simulink model "Model1_Scenario2_Faulty_2020a_35"  (R2024a)
settings: Solver=FixedStepAuto  StartTime=0.0  StopTime=300  FixedStep=1e-2  RelTol=1e-3  EnableMultiTasking=on
undefined symbols (not defined in the file): sigbuilder_block
settings Model: PacingRate=0.250000  ExtModeTrigDuration=5  Creator=Arun Mistry  LastModifiedBy=airshad
settings SolverCC: AlgebraicLoopSolver=TrustRegion
settings DataIOCC: SaveFormat=Array  SaveOutput=off  SignalLogging=off  DSMLogging=off  SaveTime=off  ReturnWorkspaceOutputs=off
settings OptimizationCC: DefaultParameterBehavior=Inlined  DefaultUnderspecifiedDataType=single  EnhancedBackFolding=on  PassReuseOutputArgsAs=Individual arguments  ZeroExternalMemoryAtStartup=off  ZeroInternalMemoryAtStartup=off  MaxStackSize=64  OptimizeBlockOrder=speed  DifferentSizesBufferReuse=on  OptimizationCustomize=off  EfficientTunableParamExpr=on
settings DebuggingCC: ParameterTunabilityLossMsg=error  UnconnectedInputMsg=warning  UnconnectedOutputMsg=warning  UnconnectedLineMsg=warning
settings HardwareCC: ProdBitPerPointer=32  ProdBitPerSizeT=32  ProdBitPerPtrDiffT=32  ProdLargestAtomicInteger=Long  ProdLargestAtomicFloat=Double  ProdWordSize=32  ProdHWDeviceType=ARM Compatible->ARM Cortex
settings ModelReferenceCC: EnableRefExpFcnMdlSchedulingChecks=on
settings SFSimCC: SimParseCustomCode=off  MATLABDynamicMemAlloc=off
settings RTWCC: Description=Embedded Coder  SystemTargetFile=ert.tlc  TemplateMakefile=ert_default_tmf  Toolchain=GNU Tools for ARM Embedded Processors  GPUComputeCapability=3.5  DLArmComputeVersion=19.05
settings CodeAppCC: ForceParamTrailComments=on  IgnoreCustomStorageClasses=off  OperatorAnnotations=on  SimulinkDataObjDesc=on  SFDataObjDesc=on  InsertBlockDesc=on
settings ERTTargetCC: ERTCustomFileTemplate=example_file_process.tlc

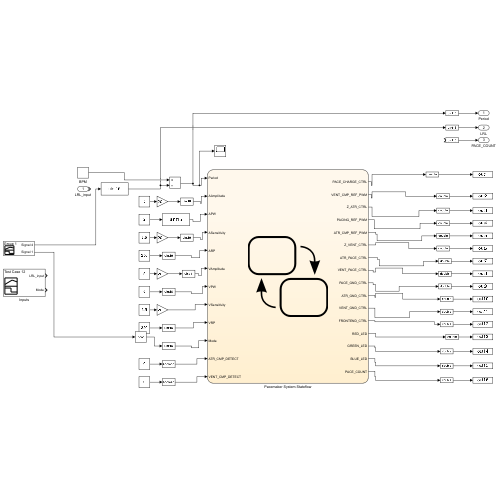
[thumbnail: Simulink's stored preview of the top-level diagram]
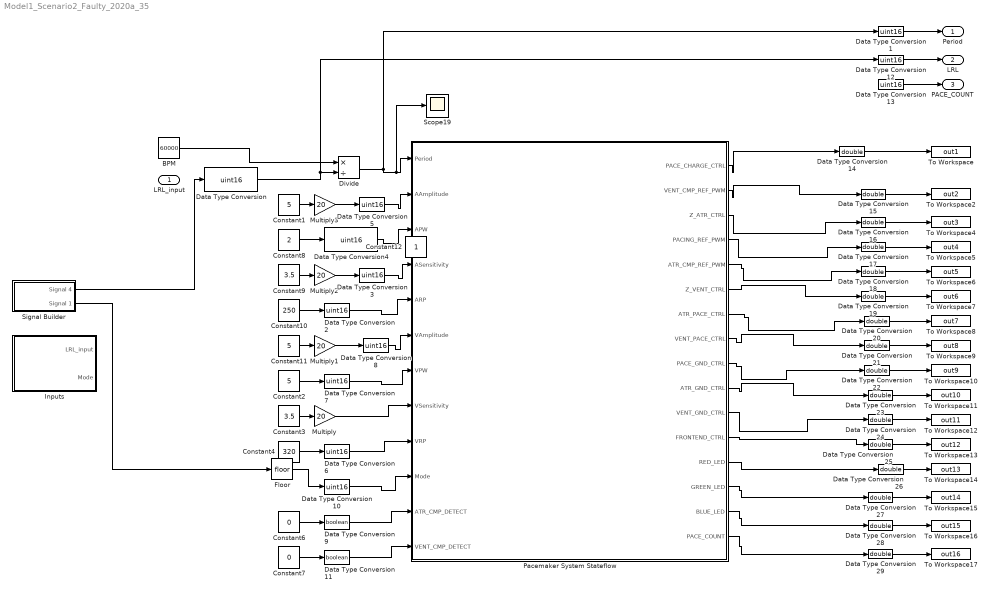
== system Model1_Scenario2_Faulty_2020a_35 ==
  LRL_input : Inport  OutDataTypeStr=double
  BPM : Constant  Value=60000
  Constant1 : Constant  Value=5
  Constant10 : Constant  Value=250
  Constant11 : Constant  Value=5
  Constant2 : Constant  Value=5
  Constant3 : Constant  Value=3.5
  Constant4 : Constant  Value=320
  Constant6 : Constant  Value=0
  Constant7 : Constant  Value=0
  Constant8 : Constant  Value=2
  Constant9 : Constant  Value=3.5
  Data Type Conversion{,1..8,10,12..13} (12 alike) : DataTypeConversion  OutDataTypeStr=uint16  SaturateOnIntegerOverflow=off  RndMeth=Floor
  Data Type Conversion11 : DataTypeConversion  OutDataTypeStr=boolean  SaturateOnIntegerOverflow=off  RndMeth=Floor
  Data Type Conversion{14..29} (16 alike) : DataTypeConversion  OutDataTypeStr=double  SaturateOnIntegerOverflow=off  RndMeth=Floor
  Data Type Conversion9 : DataTypeConversion  OutDataTypeStr=boolean  SaturateOnIntegerOverflow=off  RndMeth=Floor
  Divide : Product  Inputs=*/
  Floor : Rounding
  Inputs : Subsystem  Tag=STV Subsys  LoadFcn=sigbuilder_block('load');  StartFcn=sigbuilder_block('start');  StopFcn=sigbuilder_block('stop');  ClipboardFcn=sigbuilder_block('clipboard');  mask(Sigbuilder block){tuvar=[0:10]}
      mask init:
      | if ~strcmp(get_param(bdroot(gcb),'SimulationStatus'),'stopped'),tuvar = sigbuilder_block('maskInit'); end
      settings: CopyFcn=sigbuilder_block('copy');  DeleteFcn=sigbuilder_block('delete');  ModelCloseFcn=sigbuilder_block('modelClose');  PreSaveFcn=sigbuilder_block('preSave');  PauseFcn=sigbuilder_block('pause');  ContinueFcn=sigbuilder_block('continue');  NameChangeFcn=sigbuilder_block('namechange');  OpenFcn=sigbuilder_block('open',[50 50 520 400 ]);  CloseFcn=sigbuilder_block('close');
      mask Display: plot(0, 0, 100, 100,[2, 2, 32, 32, 2], [68, 8, 8, 68, 68],[32, 2], [38, 38], [32, 19, 2],[53, 60, 44], [32, 17, 17, 2],[16, 16, 31, 31]);txt = getActiveGroup(gcbh);text(2, 100, txt,'verticalAlignment', 'top');
  Multiply{,1..3} (4 alike) : Gain  Gain=20
  Pacemaker System Stateflow : Stateflow chart  TreatAsAtomicUnit=on
  Scope19 : Scope
  Signal Builder : Subsystem  Tag=STV Subsys  LoadFcn=sigbuilder_block('load');  StartFcn=sigbuilder_block('start');  StopFcn=sigbuilder_block('stop');  ClipboardFcn=sigbuilder_block('clipboard');  mask(Sigbuilder block){tuvar=[0:10]}
      mask help: Simulink:masks:SigbuilderBlock_MD
      mask init:
      | if ~strcmp(get_param(bdroot(gcbh),'SimulationStatus'),'stopped') tuvar = sigbuilder_block('maskInit'); end
      settings: CopyFcn=sigbuilder_block('copy');  DeleteFcn=sigbuilder_block('delete');  ModelCloseFcn=sigbuilder_block('modelClose');  PreSaveFcn=sigbuilder_block('preSave');  PauseFcn=sigbuilder_block('pause');  ContinueFcn=sigbuilder_block('continue');  NameChangeFcn=sigbuilder_block('namechange');  OpenFcn=sigbuilder_block('open',[6 26.4 948 559.8 ]);  CloseFcn=sigbuilder_block('close');
      mask Display: plot(0, 0, 100, 100,[2, 2, 32, 32, 2], [68, 8, 8, 68, 68],[32, 2], [38, 38], [32, 19, 2],[53, 60, 44], [32, 17, 17, 2],[16, 16, 31, 31]);txt = getActiveGroup(gcbh);text(2, 100, txt,'verticalAlignment', 'top');
  To Workspace : ToWorkspace  VariableName=out1  SaveFormat=Timeseries  SampleTime=-1
  To Workspace10 : ToWorkspace  VariableName=out9  SaveFormat=Timeseries  SampleTime=-1
  To Workspace11 : ToWorkspace  VariableName=out10  SaveFormat=Timeseries  SampleTime=-1
  To Workspace12 : ToWorkspace  VariableName=out11  SaveFormat=Timeseries  SampleTime=-1
  To Workspace13 : ToWorkspace  VariableName=out12  SaveFormat=Timeseries  SampleTime=-1
  To Workspace14 : ToWorkspace  VariableName=out13  SaveFormat=Timeseries  SampleTime=-1
  To Workspace15 : ToWorkspace  VariableName=out14  SaveFormat=Timeseries  SampleTime=-1
  To Workspace16 : ToWorkspace  VariableName=out15  SaveFormat=Timeseries  SampleTime=-1
  To Workspace17 : ToWorkspace  VariableName=out16  SaveFormat=Timeseries  SampleTime=-1
  To Workspace2 : ToWorkspace  VariableName=out2  SaveFormat=Timeseries  SampleTime=-1
  To Workspace4 : ToWorkspace  VariableName=out3  SaveFormat=Timeseries  SampleTime=-1
  To Workspace5 : ToWorkspace  VariableName=out4  SaveFormat=Timeseries  SampleTime=-1
  To Workspace6 : ToWorkspace  VariableName=out5  SaveFormat=Timeseries  SampleTime=-1
  To Workspace7 : ToWorkspace  VariableName=out6  SaveFormat=Timeseries  SampleTime=-1
  To Workspace8 : ToWorkspace  VariableName=out7  SaveFormat=Timeseries  SampleTime=-1
  To Workspace9 : ToWorkspace  VariableName=out8  SaveFormat=Timeseries  SampleTime=-1
  Period : Outport  OutDataTypeStr=uint16
  LRL : Outport  Port=2  OutDataTypeStr=uint16
  PACE_COUNT : Outport  Port=3
  Constant12 : Constant  IOType=siggen
  wires:
  Constant2/1 -> Data Type Conversion7/1
  Constant7/1 -> Data Type Conversion11/1
  Constant8/1 -> Data Type Conversion4/1
  Floor/1 -> Data Type Conversion10/1
  Constant10/1 -> Data Type Conversion2/1
  Multiply1/1 -> Data Type Conversion8/1
  Multiply2/1 -> Data Type Conversion3/1
  Multiply3/1 -> Data Type Conversion5/1
  Signal Builder/1(Signal 4) -> Data Type Conversion/1
  BPM/1 -> Divide/1
  Divide/1 -> Data Type Conversion1/1, Scope19/1, Pacemaker System Stateflow/1(Period)
  Pacemaker System Stateflow/1(PACE_CHARGE_CTRL) -> Data Type Conversion14/1
  Pacemaker System Stateflow/2(VENT_CMP_REF_PWM) -> Data Type Conversion15/1
  Pacemaker System Stateflow/3(Z_ATR_CTRL) -> Data Type Conversion16/1
  Pacemaker System Stateflow/4(PACING_REF_PWM) -> Data Type Conversion17/1
  Data Type Conversion/1 -> Data Type Conversion12/1, Divide/2
  Data Type Conversion1/1 -> Period/1
  Constant1/1 -> Multiply3/1
  Data Type Conversion4/1 -> Pacemaker System Stateflow/3(APW)
  Constant9/1 -> Multiply2/1
  Data Type Conversion2/1 -> Pacemaker System Stateflow/5(ARP)
  Constant6/1 -> Data Type Conversion9/1
  Data Type Conversion10/1 -> Pacemaker System Stateflow/10(Mode)
  Constant4/1 -> Data Type Conversion6/1
  Constant11/1 -> Multiply1/1
  Data Type Conversion7/1 -> Pacemaker System Stateflow/7(VPW)
  Data Type Conversion5/1 -> Pacemaker System Stateflow/2(AAmplitude)
  Data Type Conversion3/1 -> Pacemaker System Stateflow/4(ASensitivity)
  Data Type Conversion8/1 -> Pacemaker System Stateflow/6(VAmplitude)
  Constant3/1 -> Multiply/1
  Multiply/1 -> Pacemaker System Stateflow/8(VSensitivity)
  Data Type Conversion6/1 -> Pacemaker System Stateflow/9(VRP)
  Data Type Conversion11/1 -> Pacemaker System Stateflow/12(VENT_CMP_DETECT)
  Data Type Conversion9/1 -> Pacemaker System Stateflow/11(ATR_CMP_DETECT)
  Data Type Conversion12/1 -> LRL/1
  Data Type Conversion13/1 -> PACE_COUNT/1
  Signal Builder/2(Signal 1) -> Floor/1
  Pacemaker System Stateflow/5(ATR_CMP_REF_PWM) -> Data Type Conversion18/1
  Pacemaker System Stateflow/6(Z_VENT_CTRL) -> Data Type Conversion19/1
  Pacemaker System Stateflow/7(ATR_PACE_CTRL) -> Data Type Conversion20/1
  Pacemaker System Stateflow/8(VENT_PACE_CTRL) -> Data Type Conversion21/1
  Pacemaker System Stateflow/9(PACE_GND_CTRL) -> Data Type Conversion22/1
  Pacemaker System Stateflow/10(ATR_GND_CTRL) -> Data Type Conversion23/1
  Pacemaker System Stateflow/11(VENT_GND_CTRL) -> Data Type Conversion24/1
  Pacemaker System Stateflow/12(FRONTEND_CTRL) -> Data Type Conversion25/1
  Pacemaker System Stateflow/13(RED_LED) -> Data Type Conversion26/1
  Pacemaker System Stateflow/14(GREEN_LED) -> Data Type Conversion27/1
  Pacemaker System Stateflow/15(BLUE_LED) -> Data Type Conversion28/1
  Pacemaker System Stateflow/16(PACE_COUNT) -> Data Type Conversion29/1
  Data Type Conversion14/1 -> To Workspace/1
  Data Type Conversion15/1 -> To Workspace2/1
  Data Type Conversion16/1 -> To Workspace4/1
  Data Type Conversion17/1 -> To Workspace5/1
  Data Type Conversion18/1 -> To Workspace6/1
  Data Type Conversion19/1 -> To Workspace7/1
  Data Type Conversion20/1 -> To Workspace8/1
  Data Type Conversion21/1 -> To Workspace9/1
  Data Type Conversion22/1 -> To Workspace10/1
  Data Type Conversion23/1 -> To Workspace11/1
  Data Type Conversion24/1 -> To Workspace12/1
  Data Type Conversion25/1 -> To Workspace13/1
  Data Type Conversion26/1 -> To Workspace14/1
  Data Type Conversion27/1 -> To Workspace15/1
  Data Type Conversion28/1 -> To Workspace16/1
  Data Type Conversion29/1 -> To Workspace17/1

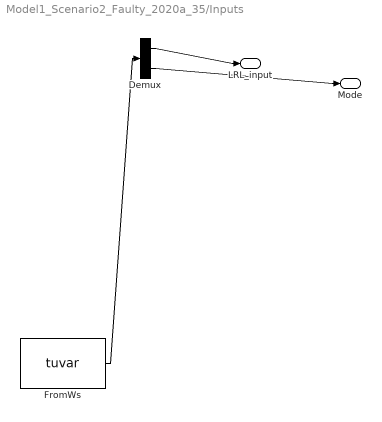
== system Model1_Scenario2_Faulty_2020a_35/Inputs ==
  Demux : Demux  Tag=STV Demux  Outputs=2
  FromWs : FromWorkspace  Tag=STV FromWs  VariableName=tuvar
      SigBuilderData=|
      | dataSet(1).timeRange = [0 0.03]
      | dataSet(1).name = 'Test Case 1'
      | dataSet(2).timeRange = [0 0.1]
      | dataSet(2).name = 'Test Case 2'
      | dataSet(3).timeRange = [0 0.1]
      | dataSet(3).name = 'Test Case 3'
      | dataSet(4).timeRange = [0 0.1]
      | dataSet(4).name = 'Test Case 4'
      | dataSet(5).timeRange = [0 0.1]
      | dataSet(5).name = 'Test Case 5'
      | dataSet(6).timeRange = [0 0.1]
      | dataSet(6).name = 'Test Case 6'
      | dataSet(7).timeRange = [0 0.1]
      | dataSet(7).name = 'Test Case 7'
      | dataSet(8).timeRange = [0 0.09]
      | dataSet(8).name = 'Test Case 8'
      | dataSet(9).timeRange = [0 0.1]
      | dataSet(9).name = 'Test Case 9'
      | dataSet(10).timeRange = [0 0.1]
      | dataSet(10).name = 'Test Case 10'
      | dataSet(11).timeRange = [0 0.09]
      | dataSet(11).name = 'Test Case 11'
      | dataSet(12).timeRange = [0 0.1]
      | dataSet(12).name = 'Test Case 12'
      | sbobj.Name = 'Signal Builder'
      | sbobj.Groups(1).Name = 'Test Case 1'
      | sbobj.Groups(1).Signals(1).Name = 'LRL_input'
      | sbobj.Groups(1).Signals(1).XData = [0 0.02 0.03]
      | sbobj.Groups(1).Signals(1).YData = [5.95663 5.95663 5.95663]
      | sbobj.Groups(1).Signals(2).Name = 'Mode'
      | sbobj.Groups(1).Signals(2).XData = [0 0.02 0.03]
      | sbobj.Groups(1).Signals(2).YData = [3 3 3]
      | sbobj.Groups(1).TimeRange = [0 0.03]
      | sbobj.Groups(2).Name = 'Test Case 2'
      | sbobj.Groups(2).Signals(1).Name = 'LRL_input'
      | sbobj.Groups(2).Signals(1).XData = [0 0.04 0.04 0.08 0.08 0.09 0.1]
      | sbobj.Groups(2).Signals(1).YData = [3.21194 3.21194 2.41404 2.41404 5.72167 5.72167 5.72167]
      | sbobj.Groups(2).Signals(2).Name = 'Mode'
      | sbobj.Groups(2).Signals(2).XData = [0 0.04 0.04 0.08 0.08 0.09 0.1]
      | sbobj.Groups(2).Signals(2).YData = [2 2 1 1 0 0 0]
      | sbobj.Groups(2).TimeRange = [0 0.1]
      | sbobj.Groups(3).Name = 'Test Case 3'
      | sbobj.Groups(3).Signals(1).Name = 'LRL_input'
      | sbobj.Groups(3).Signals(1).XData = [0 0.04 0.04 0.07 0.07 0.09 0.1]
      | sbobj.Groups(3).Signals(1).YData = [3.21194 3.21194 2.41404 2.41404 9.14622 9.14622 9.14622]
      | sbobj.Groups(3).Signals(2).Name = 'Mode'
      | sbobj.Groups(3).Signals(2).XData = [0 0.04 0.04 0.07 0.07 0.09 0.1]
      | sbobj.Groups(3).Signals(2).YData = [2 2 1 1 4 4 4]
      | sbobj.Groups(3).TimeRange = [0 0.1]
      | sbobj.Groups(4).Name = 'Test Case 4'
      | sbobj.Groups(4).Signals(1).Name = 'LRL_input'
      | sbobj.Groups(4).Signals(1).XData = [0 0.05 0.05 0.08 0.08 0.09 0.1]
      | sbobj.Groups(4).Signals(1).YData = [3.21194 3.21194 -6.6856 -6.6856 -2.71171 -2.71171 -2.71171]
      | sbobj.Groups(4).Signals(2).Name = 'Mode'
      | sbobj.Groups(4).Signals(2).XData = [0 0.05 0.05 0.08 0.08 0.09 0.1]
      | sbobj.Groups(4).Signals(2).YData = [2 2 0 0 2 2 2]
      | sbobj.Groups(4).TimeRange = [0 0.1]
      | sbobj.Groups(5).Name = 'Test Case 5'
      | sbobj.Groups(5).Signals(1).Name = 'LRL_input'
      | sbobj.Groups(5).Signals(1).XData = [0 0.05 0.05 0.09 0.1]
      | sbobj.Groups(5).Signals(1).YData = [3.21194 3.21194 -1.37522 -1.37522 -1.37522]
      | sbobj.Groups(5).Signals(2).Name = 'Mode'
      | sbobj.Groups(5).Signals(2).XData = [0 0.05 0.05 0.09 0.1]
      | sbobj.Groups(5).Signals(2).YData = [2 2 3 3 3]
      | sbobj.Groups(5).TimeRange = [0 0.1]
      | sbobj.Groups(6).Name = 'Test Case 6'
      | sbobj.Groups(6).Signals(1).Name = 'LRL_input'
      | sbobj.Groups(6).Signals(1).XData = [0 0.05 0.05 0.08 0.08 0.09 0.1]
      | sbobj.Groups(6).Signals(1).YData = [3.21194 3.21194 9.40317 9.40317 -2.04191 -2.04191 -2.04191]
      | sbobj.Groups(6).Signals(2).Name = 'Mode'
      | sbobj.Groups(6).Signals(2).XData = [0 0.05 0.05 0.08 0.08 0.09 0.1]
      | sbobj.Groups(6).Signals(2).YData = [2 2 0 0 4 4 4]
      | sbobj.Groups(6).TimeRange = [0 0.1]
      | sbobj.Groups(7).Name = 'Test Case 7'
      | sbobj.Groups(7).Signals(1).Name = 'LRL_input'
      | sbobj.Groups(7).Signals(1).XData = [0 0.05 0.05 0.08 0.08 0.09 0.1]
      | sbobj.Groups(7).Signals(1).YData = [3.21194 3.21194 -6.36929 -6.36929 -2.1928 -2.1928 -2.1928]
      | sbobj.Groups(7).Signals(2).Name = 'Mode'
      | sbobj.Groups(7).Signals(2).XData = [0 0.05 0.05 0.08 0.08 0.09 0.1]
      | sbobj.Groups(7).Signals(2).YData = [2 2 0 0 1 1 1]
      | sbobj.Groups(7).TimeRange = [0 0.1]
      | sbobj.Groups(8).Name = 'Test Case 8'
      | sbobj.Groups(8).Signals(1).Name = 'LRL_input'
      | sbobj.Groups(8).Signals(1).XData = [0 0.05 0.05 0.08 0.08 0.09]
      | sbobj.Groups(8).Signals(1).YData = [3.21194 3.21194 8.49416 8.49416 -9.92534 -9.92534]
      | sbobj.Groups(8).Signals(2).Name = 'Mode'
      | sbobj.Groups(8).Signals(2).XData = [0 0.05 0.05 0.08 0.08 0.09]
      | sbobj.Groups(8).Signals(2).YData = [2 2 4 4 2 2]
      | sbobj.Groups(8).TimeRange = [0 0.09]
      | sbobj.Groups(9).Name = 'Test Case 9'
      | sbobj.Groups(9).Signals(1).Name = 'LRL_input'
      | sbobj.Groups(9).Signals(1).XData = [0 0.02 0.02 0.05 0.05 0.09 0.1]
      | sbobj.Groups(9).Signals(1).YData = [3.21194 3.21194 7.03155 7.03155 -8.24459 -8.24459 -8.24459]
      | sbobj.Groups(9).Signals(2).Name = 'Mode'
      | sbobj.Groups(9).Signals(2).XData = [0 0.02 0.02 0.05 0.05 0.09 0.1]
      | sbobj.Groups(9).Signals(2).YData = [2 2 3 3 4 4 4]
      | sbobj.Groups(9).TimeRange = [0 0.1]
      | sbobj.Groups(10).Name = 'Test Case 10'
      | sbobj.Groups(10).Signals(1).Name = 'LRL_input'
      | sbobj.Groups(10).Signals(1).XData = [0 0.02 0.02 0.05 0.05 0.09 0.09 0.1]
      | sbobj.Groups(10).Signals(1).YData = [3.21194 3.21194 7.03155 7.03155 -8.24459 -8.24459 6.62871 6.62871]
      | sbobj.Groups(10).Signals(2).Name = 'Mode'
      | sbobj.Groups(10).Signals(2).XData = [0 0.02 0.02 0.05 0.05 0.09 0.09 0.1]
      | sbobj.Groups(10).Signals(2).YData = [2 2 3 3 4 4 2 2]
      | sbobj.Groups(10).TimeRange = [0 0.1]
      | sbobj.Groups(11).Name = 'Test Case 11'
      | sbobj.Groups(11).Signals(1).Name = 'LRL_input'
      | sbobj.Groups(11).Signals(1).XData = [0 0.05 0.05 0.08 0.08 0.09]
      | sbobj.Groups(11).Signals(1).YData = [3.21194 3.21194 -1.37522 -1.37522 -1.4663 -1.4663]
      | sbobj.Groups(11).Signals(2).Name = 'Mode'
      | sbobj.Groups(11).Signals(2).XData = [0 0.05 0.05 0.08 0.08 0.09]
      | sbobj.Groups(11).Signals(2).YData = [2 2 3 3 2 2]
      | sbobj.Groups(11).TimeRange = [0 0.09]
      | sbobj.Groups(12).Name = 'Test Case 12'
      | sbobj.Groups(12).Signals(1).Name = 'LRL_input'
      | sbobj.Groups(12).Signals(1).XData = [0 0.05 0.05 0.09 0.09 0.1]
      | sbobj.Groups(12).Signals(1).YData = [3.21194 3.21194 -1.37522 -1.37522 8.33374 8.33374]
      | sbobj.Groups(12).Signals(2).Name = 'Mode'
      | sbobj.Groups(12).Signals(2).XData = [0 0.05 0.05 0.09 0.09 0.1]
      | sbobj.Groups(12).Signals(2).YData = [2 2 3 3 2 2]
      | sbobj.Groups(12).TimeRange = [0 0.1]
  LRL_input : Outport  Tag=STV Outport
  Mode : Outport  Tag=STV Outport  Port=2
  wires:
  FromWs/1 -> Demux/1
  Demux/1 -> LRL_input/1
  Demux/2 -> Mode/1

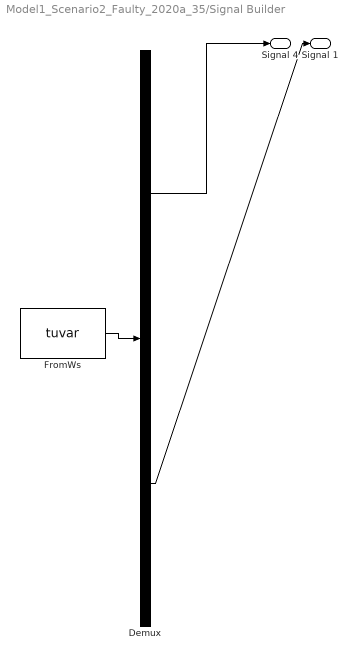
== system Model1_Scenario2_Faulty_2020a_35/Signal Builder ==
  Demux : Demux  Tag=STV Demux  Outputs=2
      settings: DisplayOption=none
  FromWs : FromWorkspace  Tag=STV FromWs  VariableName=tuvar
      SigBuilderData=|
      | common.afterFinalStr = 'Extrapolate'
      | common.sampleTime = 0
      | dataSet(1).timeRange = [0 300]
      | dataSet(1).name = 'Group 1'
      | dataSet(2).timeRange = [0 300]
      | dataSet(2).name = 'Group 2'
      | sbobj.Groups(1).Name = 'Group 1'
      | sbobj.Groups(1).Signals(1).Name = 'Signal 4'
      | sbobj.Groups(1).Signals(1).XData = [0 16.5 16.5 39.5 39.5 102 102 207 207 254.5 254.5 300]
      | sbobj.Groups(1).Signals(1).YData = [0 0 15 15 20 20 10 10 30 30 0 0]
      | sbobj.Groups(1).Signals(2).Name = 'Signal 1'
      | sbobj.Groups(1).Signals(2).XData = [0 10.5 10.5 50.5 50.5 81.5 81.5 140.5 140.5 182.5 182.5 244.5 244.5 300]
      | sbobj.Groups(1).Signals(2).YData = [0 0 4 4 3 3 4 4 2 2 1 1 0 0]
      | sbobj.Groups(1).TimeRange = [0 300]
      | sbobj.Groups(2).Name = 'Group 2'
      | sbobj.Groups(2).Signals(1).Name = 'Signal 4'
      | sbobj.Groups(2).Signals(1).XData = [0 16.5 16.5 39.5 39.5 102 102 207 254.5 300]
      | sbobj.Groups(2).Signals(1).YData = [0 0 15 15 20 20 0 0 0 0]
      | sbobj.Groups(2).Signals(2).Name = 'Signal 1'
      | sbobj.Groups(2).Signals(2).XData = [0 10.5 10.5 50.5 50.5 81.5 81.5 140.5 140.5 182.5 182.5 244.5 244.5 300]
      | sbobj.Groups(2).Signals(2).YData = [0 0 4 4 3 3 0 0 2 2 1 1 2 2]
      | sbobj.Groups(2).TimeRange = [0 300]
  Signal 4 : Outport  Tag=STV Outport
  Signal 1 : Outport  Tag=STV Outport  Port=2
  wires:
  FromWs/1 -> Demux/1
  Demux/1 -> Signal 4/1
  Demux/2 -> Signal 1/1

== stateflow chart Model1_Scenario2_Faulty_2020a_35/Pacemaker System Stateflow ==
  state AOO
    entry: % Initialize pin assigments that do not change during the states
    VENT_PACE_CTRL = 0; VENT_GND_CTRL = 0; PACE_GND_CTRL = 1;
    Z_VENT_CTRL = 0; Z_ATR_CTRL = 0;
    PACING_REF_PWM = AAmplitude; PACE_COUNT = 0;
    state PACE_ATR
      entry:
      % STOP CHARGING C22
      PACE_CHARGE_CTRL = 0;
      % DISCHARGE C22 THROUGH ATR
      ATR_GND_CTRL = 0;
      ATR_PACE_CTRL = 1;
      % PULSING INDICATOR
      BLUE_LED = 1;
      PACE_COUNT = PACE_COUNT + 1;
    state CHARGE_CAPACITOR
      entry:
      % DISCONNECT ATRIAL PACING
      ATR_PACE_CTRL = 0;
      % DISCONNECT C21 FROM GND (allow charge buildup)
      ATR_GND_CTRL = 1;
      % CHARGING C22
      PACE_CHARGE_CTRL = 1;
      % DISABLE PULSING INDICATOR
      BLUE_LED = 0;
    (default) -> AOO.CHARGE_CAPACITOR
    AOO.PACE_ATR -> AOO.CHARGE_CAPACITOR : after(APW,msec)
    AOO.CHARGE_CAPACITOR -> AOO.PACE_ATR : after(Period - 60*APW,msec)
  state MODE_ROUTER
    entry: % Reset these pins when swithching between states
    FRONTEND_CTRL = 1;
    ATR_PACE_CTRL = 0;
    ATR_GND_CTRL = 0;
    VENT_GND_CTRL = 0;
    VENT_PACE_CTRL = 0;
    Z_ATR_CTRL = 0;
    Z_VENT_CTRL = 0;
    GREEN_LED = 0;
    RED_LED = 0;
    BLUE_LED = 0;
  state VOO
    entry: % Initialize pin assigments that do not change during the states
    ATR_PACE_CTRL = 0; ATR_GND_CTRL = 0; PACE_GND_CTRL = 1;
    Z_ATR_CTRL = 0; Z_VENT_CTRL = 0; PACING_REF_PWM = VAmplitude;
    state PACE_VENT
      entry:
      % STOP CHARGING C22
      PACE_CHARGE_CTRL = 0;
      % DISCHARGE C22 THROUGH VENT
      VENT_GND_CTRL = 0;
      VENT_PACE_CTRL = 1;
      % PULSING INDICATOR
      BLUE_LED = 1;
    state CHARGE_CAPACITOR
      entry:
      % DISCONNECT VENT PACING
      VENT_PACE_CTRL = 0;
      % DISCONNECT C21 FROM GND (allow charge to buildup)
      VENT_GND_CTRL = 1;
      % CHARGING C22
      PACE_CHARGE_CTRL = 1;
      % DISABLE PULSING INDICATOR
      BLUE_LED = 0;
    (default) -> VOO.CHARGE_CAPACITOR
    VOO.PACE_VENT -> VOO.CHARGE_CAPACITOR : after(VPW,msec)
    VOO.CHARGE_CAPACITOR -> VOO.PACE_VENT : after(Period-VPW,msec)
  state AAI
    % Initialize pin assignments that do not change during the states
    entry: VENT_PACE_CTRL = 0; VENT_GND_CTRL = 0; PACE_GND_CTRL = 1;
    Z_VENT_CTRL = 0; Z_ATR_CTRL = 0; FRONTEND_CTRL = 1;
    PACING_REF_PWM = AAmplitude; ATR_CMP_REF_PWM=ASensitivity;
    state PACE_ATR
      entry:
      % STOP CHARGING C22
      PACE_CHARGE_CTRL = 0;
      % DISCHARGE C22 THROUGH ATR
      ATR_PACE_CTRL = 1;
      ATR_GND_CTRL = 0;
      % PULSING INDICATOR
      BLUE_LED = 1;
    state C22_CHARGE
      entry:
      % DISCONNECT VENT PACING
      ATR_PACE_CTRL = 0;
      % DISCONNECT C21 FROM GND (allow charge to buildup)
      ATR_GND_CTRL = 1;
      % CHARGING C22
      PACE_CHARGE_CTRL = 1;
    state REFRACTORY_STATE
      % DISABLE PULSING INDICATORS
      entry: BLUE_LED = 0; PACE_CHARGE_CTRL = 1;
      ATR_PACE_CTRL = 0;  ATR_GND_CTRL = 1;
      % DISABLE INHIBIT INIDCATOR ON EXIT
      exit: GREEN_LED = 0;
    (default) -> C22_CHARGE
    C22_CHARGE -> AAI.PACE_ATR [order 2] : after(Period - ARP, msec)
    C22_CHARGE -> REFRACTORY_STATE [order 1] : [ATR_CMP_DETECT]
        | {GREEN_LED = 1}
    REFRACTORY_STATE -> C22_CHARGE : after(ARP, msec)
    AAI.PACE_ATR -> REFRACTORY_STATE : after(APW, msec)
  state VVI
    % Initialize pin assignments that do not change during the states
    entry: ATR_PACE_CTRL = 0; ATR_GND_CTRL = 0; PACE_GND_CTRL = 1;
    Z_VENT_CTRL = 0; Z_ATR_CTRL = 0; FRONTEND_CTRL = 1;
    PACING_REF_PWM = VAmplitude; VENT_CMP_REF_PWM = VSensitivity;
    state PACE_VENT
      entry:
      % STOP CHARGING C22
      PACE_CHARGE_CTRL = 0;
      % DISCHARGE C22 THROUGH VENT
      VENT_PACE_CTRL = 1;
      VENT_GND_CTRL = 0;
      % PULSING INDICATOR
      BLUE_LED = 1;
    state CHARGE_CAPACITOR
      entry:
      % CHARGING C22
      PACE_CHARGE_CTRL = 1;
      % DISCONNECT VENT PACING
      VENT_PACE_CTRL = 0;
      % DISCONNECT FROM GND
      VENT_GND_CTRL = 1;
    state REFRACTORY
      % DISABLE PULSING INDICATOR
      entry: BLUE_LED = 0; PACE_CHARGE_CTRL = 1;
      VENT_PACE_CTRL = 0;  VENT_GND_CTRL = 1;
      % DISABLE INHIBIT INDICATOR ON EXIT (if on)
      exit: GREEN_LED = 0;
    (default) -> VVI.CHARGE_CAPACITOR
    VVI.CHARGE_CAPACITOR -> VVI.PACE_VENT [order 2] : after(Period - VRP, msec)
    VVI.CHARGE_CAPACITOR -> REFRACTORY [order 1] : [VENT_CMP_DETECT]
        | {GREEN_LED = 1}
    REFRACTORY -> VVI.CHARGE_CAPACITOR : after(VRP, msec)
    VVI.PACE_VENT -> REFRACTORY : after(VPW, msec)
  (default) -> MODE_ROUTER
  MODE_ROUTER -> VOO [order 2] : [Mode==2]
  MODE_ROUTER -> AOO [order 1] : [Mode==1]
  VOO -> MODE_ROUTER : [Mode~=2]
  AOO -> MODE_ROUTER : [Mode~=1]
  MODE_ROUTER -> AAI [order 3] : [Mode==3]
  MODE_ROUTER -> VVI [order 4] : [Mode==4]
  AAI -> MODE_ROUTER : [Mode~=3]
  VVI -> MODE_ROUTER : [Mode~=4]
  data: Period input double; AAmplitude input uint16; APW input uint16; ASensitivity input uint16; ARP input uint16; VAmplitude input uint16; VPW input uint16; VSensitivity input double; VRP input uint16; PACE_CHARGE_CTRL output double; VENT_CMP_REF_PWM output double; Z_ATR_CTRL output double; PACING_REF_PWM output uint16; ATR_CMP_REF_PWM output uint16; Z_VENT_CTRL output uint16; ATR_PACE_CTRL output uint16; VENT_PACE_CTRL output uint16; PACE_GND_CTRL output uint16; ATR_GND_CTRL output uint16; VENT_GND_CTRL output uint16; Mode input uint16; FRONTEND_CTRL output uint16; RED_LED output uint16; GREEN_LED output uint16; BLUE_LED output uint16; ATR_CMP_DETECT input boolean; VENT_CMP_DETECT input boolean; PACE_COUNT output
